simulink model "q3"  (Simulink 9.3)
settings: Solver=FixedStepAuto  StartTime=0.0  StopTime=1.5  FixedStep=2e-7  RelTol=1e-3
libraries: dsparch4 x2, simulink x2
settings Model: Creator=marco  LastModifiedBy=marco
settings DataIOCC: SaveFormat=Dataset  SignalLoggingSaveFormat=Dataset  ReturnWorkspaceOutputs=on
settings OptimizationCC: LifeSpan=auto
settings DebuggingCC: UnderspecifiedInitializationDetection=Simplified  MergeDetectMultiDrivingBlocksExec=error  FcnCallInpInsideContextMsg=error  SFUnexpectedBacktrackingDiag=error  SFNoUnconditionalDefaultTransitionDiag=error  SFExecutionAtInitializationDiag=warning  ArithmeticOperatorsInVariantConditions=error
settings HardwareCC: ProdBitPerPointer=64  ProdBitPerSizeT=64  ProdBitPerPtrDiffT=64  ProdLargestAtomicFloat=Float  ProdIntDivRoundTo=Zero  ProdEndianess=LittleEndian  ProdWordSize=64  ProdHWDeviceType=Intel->x86-64 (Windows64)
settings ModelReferenceCC: PropagateSignalLabelsOutOfModel=on
settings SFSimCC: SimUseLocalCustomCode=on
settings RTWCC: RTWUseLocalCustomCode=on
settings CodeAppCC: StateflowObjectComments=off
settings GRTTargetCC: TargetLangStandard=C99 (ISO)  CombineOutputUpdateFcns=on  GRTInterface=off
settings ConfigComp: CovMetricSettings=dwe  CovHtmlReporting=off  CovSaveCumulativeToWorkspaceVar=off  CovSaveSingleToWorkspaceVar=off  CovExternalEMLEnable=on

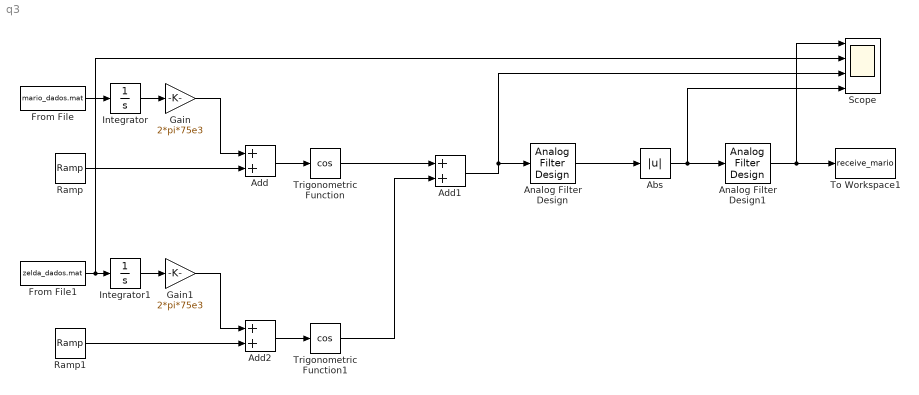
== system q3 ==
  Abs : Abs
  Add : Sum
  Add1 : Sum
  Add2 : Sum
  Analog Filter Design : dsparch4/Analog Filter Design  method=Butterworth  filttype=Bandpass  N=8  Wlo=2*pi*(1150e3 - 50e3)  Whi=2*pi*(1150e3 + 50e3)  Rp=2  Rs=40
  Analog Filter Design1 : dsparch4/Analog Filter Design  method=Butterworth  filttype=Lowpass  N=8  Wlo=2*pi*200e3  Whi=80  Rp=2  Rs=40
  From File : FromFile  FileName=mario_dados.mat  SampleTime=0  ExtrapolationBeforeFirstDataPoint=Ground value
  From File1 : FromFile  FileName=zelda_dados.mat  SampleTime=0  ExtrapolationBeforeFirstDataPoint=Ground value
  Gain : Gain  Gain=2*pi*75e3
  Gain1 : Gain  Gain=2*pi*75e3
  Integrator : Integrator
  Integrator1 : Integrator
  Ramp : simulink/Sources/Ramp  slope=2*pi*(950e3)  start=0  InitialOutput=0
  Ramp1 : simulink/Sources/Ramp  slope=2*pi*(1050e3)  start=0  InitialOutput=0
  Scope : Scope  NumInputPorts=4
  To Workspace1 : ToWorkspace  VariableName=receive_mario  SaveFormat=Timeseries  SampleTime=1e-5
  Trigonometric Function : Trigonometry  Operator=cos
  Trigonometric Function1 : Trigonometry  Operator=cos
  wires:
  Add/1 -> Trigonometric Function/1
  Ramp/1 -> Add/2
  From File/1 -> Integrator/1
  Integrator/1 -> Gain/1
  Gain/1 -> Add/1
  Analog Filter Design/1 -> Abs/1
  Abs/1 -> Scope/4, Analog Filter Design1/1
  Analog Filter Design1/1 -> To Workspace1/1, Scope/1
  Trigonometric Function/1 -> Add1/1
  Add1/1 -> Scope/3, Analog Filter Design/1
  Add2/1 -> Trigonometric Function1/1
  Gain1/1 -> Add2/1
  Integrator1/1 -> Gain1/1
  From File1/1 -> Scope/2, Integrator1/1
  Ramp1/1 -> Add2/2
  Trigonometric Function1/1 -> Add1/2
